simulink model "untitled"  (R2015b)
settings: Solver=VariableStepAuto  StartTime=0.0  StopTime=2  RelTol=1e-3
values from neighbouring files (symbols this model uses):
  bHI = 35    [Initiation.m]
  bWall = 0    [Initiation.m]    (also in VirtualEnvironment.m = block.DialogPrm(2).Data; Virtual_Environment.m = block.DialogPrm(2).Data)
  kWall = 90000    [Initiation.m]    (also in VirtualEnvironment.m = block.DialogPrm(1).Data; Virtual_Environment.m = block.DialogPrm(1).Data)
  m = 1    [Initiation.m]
  nWall = 1    [Initiation.m]    (also in VirtualEnvironment.m = block.DialogPrm(3).Data; Virtual_Environment.m = block.DialogPrm(3).Data)
  tsampling = 0.001    [Initiation.m]    (also in VirtualEnvironment.m = block.DialogPrm(6).Data; Virtual_Environment.m = block.DialogPrm(6).Data)
  x0 = 0.14    [Initiation.m]    (also in PC.m = []; Wall.m = []; devision.m = []; sgn.m = [])
  x_dot0 = 0    [Initiation.m]
  xWall = 0.085    [Initiation.m]
undefined symbols (not defined in the file or in its folder): DiscIntNeverNeededParam
libraries: simulink x3
settings Model: Creator=TOSHIBA  LastModifiedBy=TOSHIBA

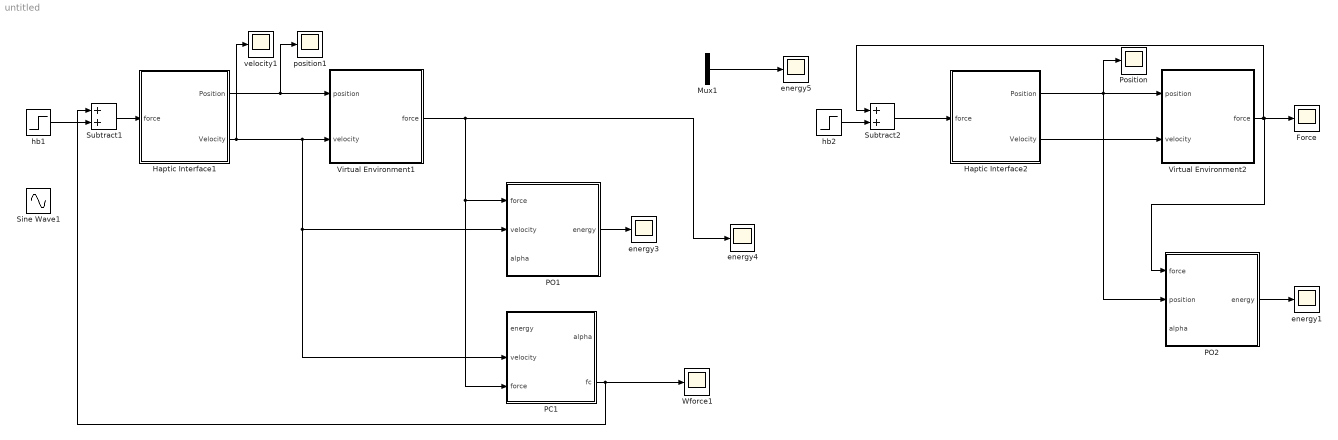
== system untitled ==
  Force : Scope
  Haptic Interface1 : Subsystem
  Haptic Interface2 : Subsystem
  Mux1 : Mux
  PC1 : Subsystem
  PO1 : Subsystem
  PO2 : Subsystem
  Position : Scope
  Sine Wave1 : Sin  Frequency=pi  Phase=pi/2  SampleTime=0
  Subtract1 : Sum
  Subtract2 : Sum
  Virtual Environment1 : Subsystem
  Virtual Environment2 : Subsystem
  Wforce1 : Scope
  energy{1,3..5} (4 alike) : Scope
  hb1 : Step  Time=0.35  After=-10  SampleTime=0
  hb2 : Step  Time=0.7  After=-5  SampleTime=0
  position1 : Scope
  velocity1 : Scope
  wires:
  Subtract1/1 -> Haptic Interface1/1(force)
  Haptic Interface1/1(Position) -> position1/1, Virtual Environment1/1(position)
  hb1/1 -> Subtract1/2
  Mux1/1 -> energy5/1
  Haptic Interface1/2(Velocity) -> velocity1/1, PC1/2(velocity), PO1/2(velocity), Virtual Environment1/2(velocity)
  PO1/1(energy) -> energy3/1
  Virtual Environment1/1(force) -> PC1/3(force), PO1/1(force), energy4/1
  PC1/2(fc) -> Wforce1/1, Subtract1/1
  Haptic Interface2/1(Position) -> Position/1, PO2/2(position), Virtual Environment2/1(position)
  Haptic Interface2/2(Velocity) -> Virtual Environment2/2(velocity)
  Virtual Environment2/1(force) -> Force/1, PO2/1(force), Subtract2/1
  hb2/1 -> Subtract2/2
  Subtract2/1 -> Haptic Interface2/1(force)
  PO2/1(energy) -> energy1/1

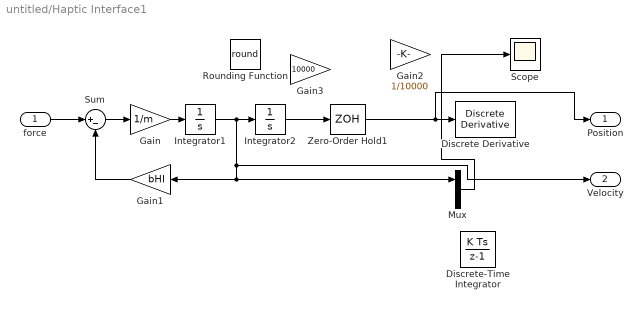
== system untitled/Haptic Interface1 ==
  force : Inport
  Discrete Derivative : simulink/Discrete/Discrete Derivative  gainval=1.0  ICPrevScaledInput=x0  InputProcessing=Inherited  OutMin=[]  OutMax=[]  OutDataType=fixdt(1, 16)  OutScaling=2^-10  DoSatur=off
  Discrete-Time Integrator : DiscreteIntegrator  InitialCondition=x0  InitialConditionSetting=State (most efficient)  SampleTime=tsampling  ICPrevOutput=DiscIntNeverNeededParam  ICPrevScaledInput=DiscIntNeverNeededParam
  Gain : Gain  Gain=1/m
  Gain1 : Gain  Gain=bHI
  Gain2 : Gain  Gain=1/10000
  Gain3 : Gain  Gain=10000
  Integrator1 : Integrator  InitialCondition=x_dot0
  Integrator2 : Integrator  InitialCondition=x0
  Mux : Mux  Inputs=2
  Rounding Function : Rounding  Operator=round
  Scope : Scope
  Sum : Sum  Inputs=|+-
  Zero-Order Hold1 : ZeroOrderHold  SampleTime=tsampling
  Position : Outport
  Velocity : Outport  Port=2
  wires:
  Gain1/1 -> Sum/2
  Integrator1/1 -> Mux/1, Gain1/1, Velocity/1, Integrator2/1
  Gain/1 -> Integrator1/1
  force/1 -> Sum/1
  Sum/1 -> Gain/1
  Zero-Order Hold1/1 -> Position/1, Discrete Derivative/1
  Mux/1 -> Scope/1
  Integrator2/1 -> Zero-Order Hold1/1

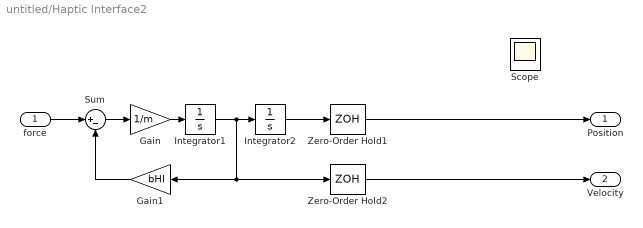
== system untitled/Haptic Interface2 ==
  force : Inport
  Gain : Gain  Gain=1/m
  Gain1 : Gain  Gain=bHI
  Integrator1 : Integrator  InitialCondition=x_dot0
  Integrator2 : Integrator  InitialCondition=x0
  Scope : Scope
  Sum : Sum  Inputs=|+-
  Zero-Order Hold1 : ZeroOrderHold  SampleTime=tsampling
  Zero-Order Hold2 : ZeroOrderHold  SampleTime=tsampling
  Position : Outport
  Velocity : Outport  Port=2
  wires:
  Integrator2/1 -> Zero-Order Hold1/1
  Sum/1 -> Gain/1
  force/1 -> Sum/1
  Gain/1 -> Integrator1/1
  Integrator1/1 -> Integrator2/1, Zero-Order Hold2/1, Gain1/1
  Gain1/1 -> Sum/2
  Zero-Order Hold2/1 -> Velocity/1
  Zero-Order Hold1/1 -> Position/1

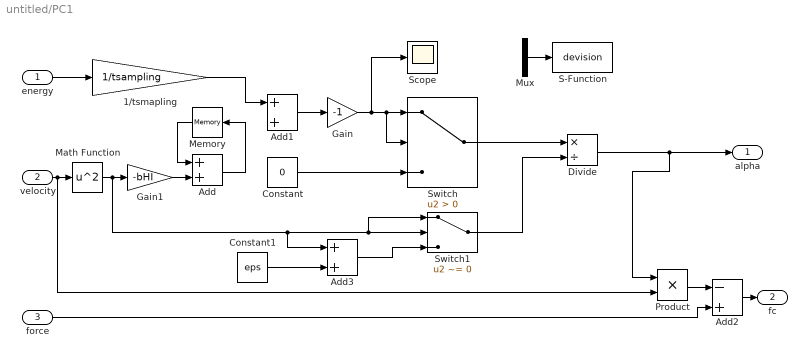
== system untitled/PC1 ==
  energy : Inport
  velocity : Inport  Port=2
  force : Inport  Port=3
  1/tsmapling : Gain  Gain=1/tsampling
  Add : Sum
  Add1 : Sum
  Add2 : Sum  Inputs=-+
  Add3 : Sum
  Constant : Constant  Value=0
  Constant1 : Constant  Value=eps
  Divide : Product  Inputs=*/
  Gain : Gain  Gain=-1
  Gain1 : Gain  Gain=-bHI
  Math Function : Math  Operator=square  SaturateOnIntegerOverflow=on
  Memory : Memory
  Mux : Mux  Inputs=2
  Product : Product
  S-Function : S-Function  FunctionName=devision  Parameters=tsampling  SFunctionDeploymentMode=off  EnableBusSupport=off
  Scope : Scope
  Switch : Switch  Criteria=u2 > Threshold
  Switch1 : Switch  Criteria=u2 ~= 0
  alpha : Outport
  fc : Outport  Port=2
  wires:
  Add/1 -> Memory/1
  Add1/1 -> Gain/1
  Memory/1 -> Add/1
  Gain1/1 -> Add/2
  Math Function/1 -> Add3/1, Switch1/1, Switch1/2, Gain1/1
  velocity/1 -> Product/2, Math Function/1
  1/tsmapling/1 -> Add1/1
  energy/1 -> 1/tsmapling/1
  Constant/1 -> Switch/3
  Gain/1 -> Switch/1, Switch/2, Scope/1
  force/1 -> Add2/2
  Product/1 -> Add2/1
  Add2/1 -> fc/1
  Mux/1 -> S-Function/1
  Switch/1 -> Divide/1
  Divide/1 -> Product/1, alpha/1
  Switch1/1 -> Divide/2
  Add3/1 -> Switch1/3
  Constant1/1 -> Add3/2

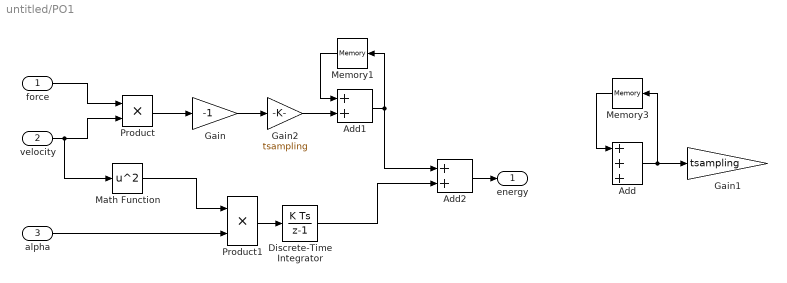
== system untitled/PO1 ==
  force : Inport
  velocity : Inport  Port=2
  alpha : Inport  Port=3
  Add : Sum  Inputs=+++
  Add1 : Sum
  Add2 : Sum
  Discrete-Time Integrator : DiscreteIntegrator  InitialConditionSetting=State (most efficient)  SampleTime=tsampling  ICPrevOutput=DiscIntNeverNeededParam  ICPrevScaledInput=DiscIntNeverNeededParam
  Gain : Gain  Gain=-1
  Gain1 : Gain  Gain=tsampling
  Gain2 : Gain  Gain=tsampling
  Math Function : Math  Operator=square  SaturateOnIntegerOverflow=on
  Memory1 : Memory
  Memory3 : Memory
  Product : Product
  Product1 : Product
  energy : Outport
  wires:
  alpha/1 -> Product1/2
  Math Function/1 -> Product1/1
  Memory3/1 -> Add/1
  Product1/1 -> Discrete-Time Integrator/1
  Add/1 -> Gain1/1, Memory3/1
  Product/1 -> Gain/1
  velocity/1 -> Product/2, Math Function/1
  force/1 -> Product/1
  Add1/1 -> Memory1/1, Add2/1
  Gain/1 -> Gain2/1
  Memory1/1 -> Add1/1
  Gain2/1 -> Add1/2
  Add2/1 -> energy/1
  Discrete-Time Integrator/1 -> Add2/2

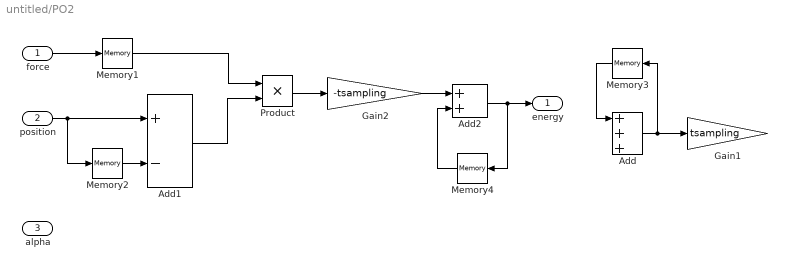
== system untitled/PO2 ==
  force : Inport
  position : Inport  Port=2
  alpha : Inport  Port=3
  Add : Sum  Inputs=+++
  Add1 : Sum  Inputs=+-
  Add2 : Sum
  Gain1 : Gain  Gain=tsampling
  Gain2 : Gain  Gain=-tsampling
  Memory{1..4} (4 alike) : Memory
  Product : Product
  energy : Outport
  wires:
  Add2/1 -> Memory4/1, energy/1
  Add/1 -> Memory3/1, Gain1/1
  Memory3/1 -> Add/1
  force/1 -> Memory1/1
  position/1 -> Memory2/1, Add1/1
  Memory2/1 -> Add1/2
  Memory1/1 -> Product/1
  Add1/1 -> Product/2
  Product/1 -> Gain2/1
  Gain2/1 -> Add2/1
  Memory4/1 -> Add2/2

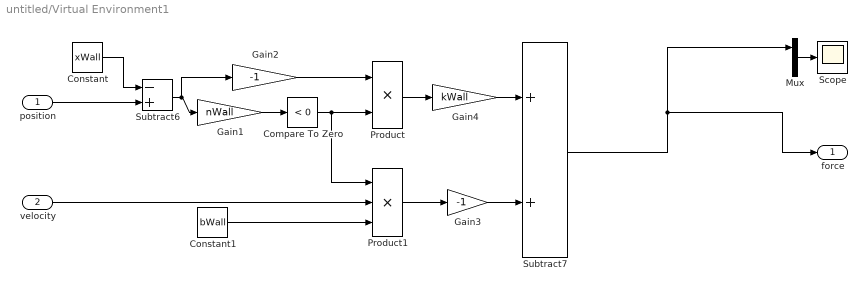
== system untitled/Virtual Environment1 ==
  position : Inport
  velocity : Inport  Port=2
  Compare To Zero : simulink/Logic and Bit Operations/Compare To Zero  relop=<  OutDataTypeStr=boolean
  Constant : Constant  Value=xWall
  Constant1 : Constant  Value=bWall
  Gain1 : Gain  Gain=nWall
  Gain2 : Gain  Gain=-1
  Gain3 : Gain  Gain=-1
  Gain4 : Gain  Gain=kWall
  Mux : Mux  Inputs=2
  Product : Product
  Product1 : Product  Inputs=3
  Scope : Scope
  Subtract6 : Sum  Inputs=-+
  Subtract7 : Sum
  force : Outport
  wires:
  velocity/1 -> Product1/2
  Gain3/1 -> Subtract7/2
  Constant1/1 -> Product1/3
  Product1/1 -> Gain3/1
  position/1 -> Subtract6/2
  Gain1/1 -> Compare To Zero/1
  Compare To Zero/1 -> Product/2, Product1/1
  Product/1 -> Gain4/1
  Gain4/1 -> Subtract7/1
  Gain2/1 -> Product/1
  Constant/1 -> Subtract6/1
  Subtract6/1 -> Gain1/1, Gain2/1
  Subtract7/1 -> force/1, Mux/1
  Mux/1 -> Scope/1

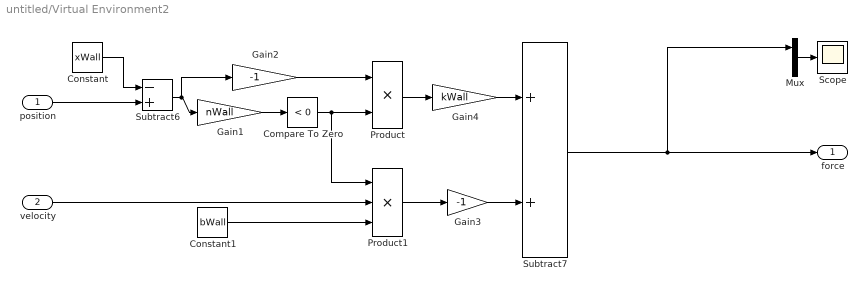
== system untitled/Virtual Environment2 ==
  position : Inport
  velocity : Inport  Port=2
  Compare To Zero : simulink/Logic and Bit Operations/Compare To Zero  relop=<  OutDataTypeStr=boolean
  Constant : Constant  Value=xWall
  Constant1 : Constant  Value=bWall
  Gain1 : Gain  Gain=nWall
  Gain2 : Gain  Gain=-1
  Gain3 : Gain  Gain=-1
  Gain4 : Gain  Gain=kWall
  Mux : Mux  Inputs=2
  Product : Product
  Product1 : Product  Inputs=3
  Scope : Scope
  Subtract6 : Sum  Inputs=-+
  Subtract7 : Sum
  force : Outport
  wires:
  Mux/1 -> Scope/1
  Subtract7/1 -> Mux/1, force/1
  Subtract6/1 -> Gain2/1, Gain1/1
  Constant/1 -> Subtract6/1
  Gain2/1 -> Product/1
  Gain4/1 -> Subtract7/1
  Product/1 -> Gain4/1
  Compare To Zero/1 -> Product1/1, Product/2
  Gain1/1 -> Compare To Zero/1
  position/1 -> Subtract6/2
  Product1/1 -> Gain3/1
  Constant1/1 -> Product1/3
  Gain3/1 -> Subtract7/2
  velocity/1 -> Product1/2
